simulink library "Animation_Lib"  (R2022b)
settings: Solver=ode45  StartTime=0.0  StopTime=10.0  RelTol=1e-3  EnableMultiTasking=on
undefined symbols (not defined in the file or in its folder): DCT_Param
libraries: vrlib x5, simulink x2, $bdroot x1
Description:
  | Copyright 2014-2022 The MathWorks, Inc.
settings Model: Creator=smiller  LastModifiedBy=smiller
settings SolverCC: AlgebraicLoopSolver=TrustRegion
settings DataIOCC: LimitDataPoints=on  SaveFormat=Array  SignalLoggingSaveFormat=ModelDataLogs  ReturnWorkspaceOutputs=off
settings OptimizationCC: ExpressionDepthLimit=2147483647  LifeSpan=inf
settings DebuggingCC: UnderspecifiedInitializationDetection=Classic  MergeDetectMultiDrivingBlocksExec=none  SolverPrmCheckMsg=warning  FcnCallInpInsideContextMsg=warning  UnconnectedInputMsg=warning  UnconnectedOutputMsg=warning  UnconnectedLineMsg=warning  AllowSymbolicDim=off  StateNameClashWarn=warning  PregeneratedLibrarySubsystemCodeDiagnostic=none  SFUnexpectedBacktrackingDiag=warning  SFNoUnconditionalDefaultTransitionDiag=warning  SFExecutionAtInitializationDiag=none  SFMachineParentedDataDiag=warning  ArithmeticOperatorsInVariantConditions=warning
settings HardwareCC: ProdBitPerPointer=32  ProdBitPerSizeT=32  ProdBitPerPtrDiffT=32  ProdLargestAtomicFloat=None  ProdIntDivRoundTo=Undefined  ProdEndianess=Unspecified  ProdWordSize=32  ProdHWDeviceType=32-bit Generic
settings ModelReferenceCC: EnableRefExpFcnMdlSchedulingChecks=on  PropagateSignalLabelsOutOfModel=off
settings SFSimCC: SimUseLocalCustomCode=off  CustomCodeUndefinedFunction=UseInterfaceOnly
settings RTWCC: RTWUseLocalCustomCode=off  DLArmComputeVersion=19.05
settings CodeAppCC: StateflowObjectComments=on
settings GRTTargetCC: TargetLangStandard=C89/C90 (ANSI)  CombineOutputUpdateFcns=off  GRTInterface=on
settings ConfigComp: CovMetricSettings=dw  CovSaveCumulativeToWorkspaceVar=on  CovSaveSingleToWorkspaceVar=on  CovExternalEMLEnable=off  CovSFcnEnable=off

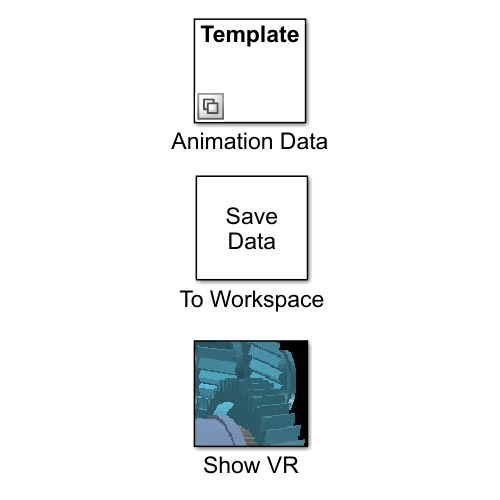
[thumbnail: Simulink's stored preview of the top-level diagram]
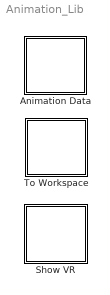
== system Animation_Lib ==
  Animation Data : Subsystem  BlockChoice=Show VR
      settings: TemplateBlock=self  MemberBlocks=Show VR,To Workspace
  Show VR : Subsystem
      mask Display: image(imread('DCT_Animation_Show_VR_IMAGE.jpg'));
  To Workspace : Subsystem
      mask Display: disp('Save\nData');

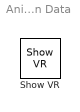
== system Animation_Lib/Animation Data ==
  Show VR : $bdroot/Show VR  SystemSampleTime=-1  VariantActivationTime=update diagram  Latency=0  AutoFrameSizeCalculation=off

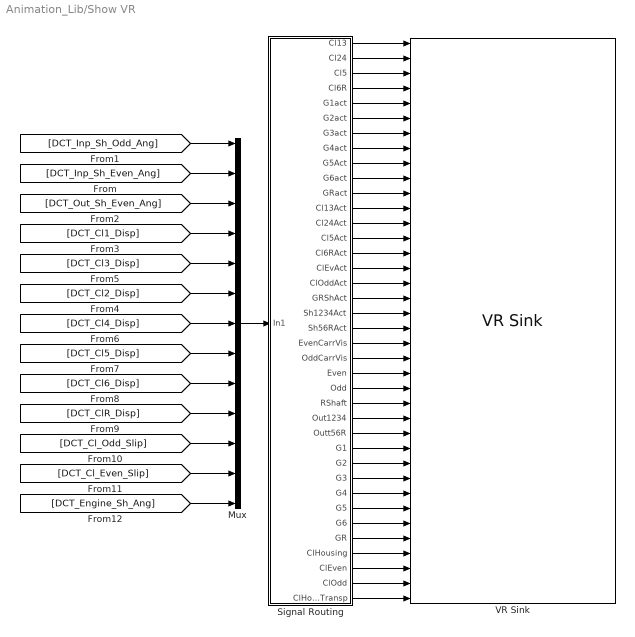
== system Animation_Lib/Show VR ==
  Mux : Mux  Inputs=13
  Signal Routing : Subsystem
  VR Sink : vrlib/VR Sink  InstantiateOnLoad=on  SampleTime=0.1  ViewEnable=on  RemoteChange=off  RemoteView=off  FieldsWritten=DCT.Selector_13_Control.1.1.1.double#DCT.Selector_24_Control.1.1.1.double#DCT.Selector_5_Control.1.1.1.double#DCT.Selector_6R_Control.1.1.1.double#DCT.Gear_1_Active.1.1.1.logical#DCT.Gear_2_Active.1.1.1.logical#DCT.Gear_3_Active.1.1.1.logical#DCT.Gear_4_Active.1.1.1.logical#DCT.Gear_5_Active.1.1.1.logical#DCT.Gear_6_Active.1.1.1.logical#DCT.Gear_R_Active.1.1.1.logical#DCT.Selector_13_Active.1.1.1.logical#DCT.Selector_24_Active.1.1.1.logical#DCT.Selector_5_Active.1.1.1.logical#DCT.Selector_6R_Active.1.1.1.logical#DCT.Clutch_Even_Active.1.1.1.logical#DCT.Clutch_Odd_Active.1.1.1.logical#DCT.Reverse_Shaft_Active.1.1.1.logical#DCT.Shaft_1234_Active.1.1.1.logical#DCT.Shaft_56R_Active.1.1.1.logical#DCT.Clutch_Even_CarrierVis.1.1.1.logical#DCT.Clutch_Odd_CarrierVis.1.1.1.logical#DCT.Input_Shaft_Even_Rot.4.1.1.double#DCT.Input_Shaft_Odd_Rot.4.1.1.double#DCT.Reverse_Shaft_Rot.4.1.1.double#DCT.Output_Shaft_1234_Rot.4.1.1.double#DCT.Output_Shaft_56R_Rot.4.1.1.double#DCT.Gear_1_Rot.4.1.1.double#DCT.Gear_2_Rot.4.1.1.double#DCT.Gear_3_Rot.4.1.1.double#DCT.Gear_4_Rot.4.1.1.double#DCT.Gear_5_Rot.4.1.1.double#DCT.Gear_6_Rot.4.1.1.double#DCT.Gear_R_Rot.4.1.1.double#DCT.Clutch_Driving_Rot.4.1.1.double#DCT.Clutch_Even_Rot.4.1.1.double#DCT.Clutch_Odd_Rot.4.1.1.double#DCT.Clutch_Transparency.1.1.1.double  WorldFileName=DCT_Gearbox_Animation.wrl  WorldDescription=Dual Clutch Transmission  AutoView=off  VideoDimensions=[]  AllowVariableSize=off
  wires:
  [DCT_Inp_Sh_Even_Ang] -> Mux/2
  [DCT_Inp_Sh_Odd_Ang] -> Mux/1
  [DCT_Out_Sh_Even_Ang] -> Mux/3
  [DCT_Cl1_Disp] -> Mux/4
  [DCT_Cl3_Disp] -> Mux/5
  [DCT_Cl2_Disp] -> Mux/6
  [DCT_Cl4_Disp] -> Mux/7
  [DCT_Cl5_Disp] -> Mux/8
  [DCT_Cl6_Disp] -> Mux/9
  [DCT_ClR_Disp] -> Mux/10
  [DCT_Cl_Odd_Slip] -> Mux/11
  [DCT_Cl_Even_Slip] -> Mux/12
  Signal Routing/22(OddCarrVis) -> VR Sink/22
  Signal Routing/21(EvenCarrVis) -> VR Sink/21
  Signal Routing/24(Odd) -> VR Sink/24
  Signal Routing/1(Cl13) -> VR Sink/1
  Signal Routing/26(Out1234) -> VR Sink/26
  Signal Routing/27(Outt56R) -> VR Sink/27
  Signal Routing/28(G1) -> VR Sink/28
  Signal Routing/29(G2) -> VR Sink/29
  Signal Routing/30(G3) -> VR Sink/30
  Signal Routing/31(G4) -> VR Sink/31
  Signal Routing/2(Cl24) -> VR Sink/2
  Signal Routing/5(G1act) -> VR Sink/5
  Signal Routing/7(G3act) -> VR Sink/7
  Signal Routing/6(G2act) -> VR Sink/6
  Signal Routing/8(G4act) -> VR Sink/8
  Signal Routing/3(Cl5) -> VR Sink/3
  Signal Routing/10(G6act) -> VR Sink/10
  Signal Routing/11(GRact) -> VR Sink/11
  Signal Routing/4(Cl6R) -> VR Sink/4
  Signal Routing/32(G5) -> VR Sink/32
  Signal Routing/12(Cl13Act) -> VR Sink/12
  Signal Routing/13(Cl24Act) -> VR Sink/13
  Signal Routing/9(G5Act) -> VR Sink/9
  Signal Routing/14(Cl5Act) -> VR Sink/14
  Signal Routing/15(Cl6RAct) -> VR Sink/15
  Signal Routing/18(GRShAct) -> VR Sink/18
  Signal Routing/16(ClEvAct) -> VR Sink/16
  Signal Routing/17(ClOddAct) -> VR Sink/17
  Signal Routing/19(Sh1234Act) -> VR Sink/19
  Signal Routing/20(Sh56RAct) -> VR Sink/20
  Signal Routing/25(RShaft) -> VR Sink/25
  Signal Routing/23(Even) -> VR Sink/23
  Signal Routing/33(G6) -> VR Sink/33
  Signal Routing/34(GR) -> VR Sink/34
  Signal Routing/35(ClHousing) -> VR Sink/35
  Signal Routing/36(ClEven) -> VR Sink/36
  Mux/1 -> Signal Routing/1(In1)
  [DCT_Engine_Sh_Ang] -> Mux/13
  Signal Routing/37(ClOdd) -> VR Sink/37
  Signal Routing/38(ClHousTransp) -> VR Sink/38

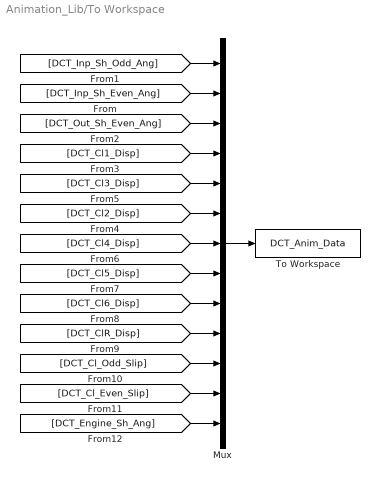
== system Animation_Lib/To Workspace ==
  Mux : Mux  Inputs=13
  To Workspace : ToWorkspace  VariableName=DCT_Anim_Data  SaveFormat=Structure With Time  SampleTime=-1
  wires:
  [DCT_Cl_Even_Slip] -> Mux/12
  [DCT_Cl_Odd_Slip] -> Mux/11
  [DCT_ClR_Disp] -> Mux/10
  [DCT_Cl6_Disp] -> Mux/9
  [DCT_Cl5_Disp] -> Mux/8
  [DCT_Cl4_Disp] -> Mux/7
  [DCT_Cl2_Disp] -> Mux/6
  [DCT_Cl3_Disp] -> Mux/5
  [DCT_Cl1_Disp] -> Mux/4
  [DCT_Out_Sh_Even_Ang] -> Mux/3
  [DCT_Inp_Sh_Odd_Ang] -> Mux/1
  [DCT_Inp_Sh_Even_Ang] -> Mux/2
  Mux/1 -> To Workspace/1
  [DCT_Engine_Sh_Ang] -> Mux/13

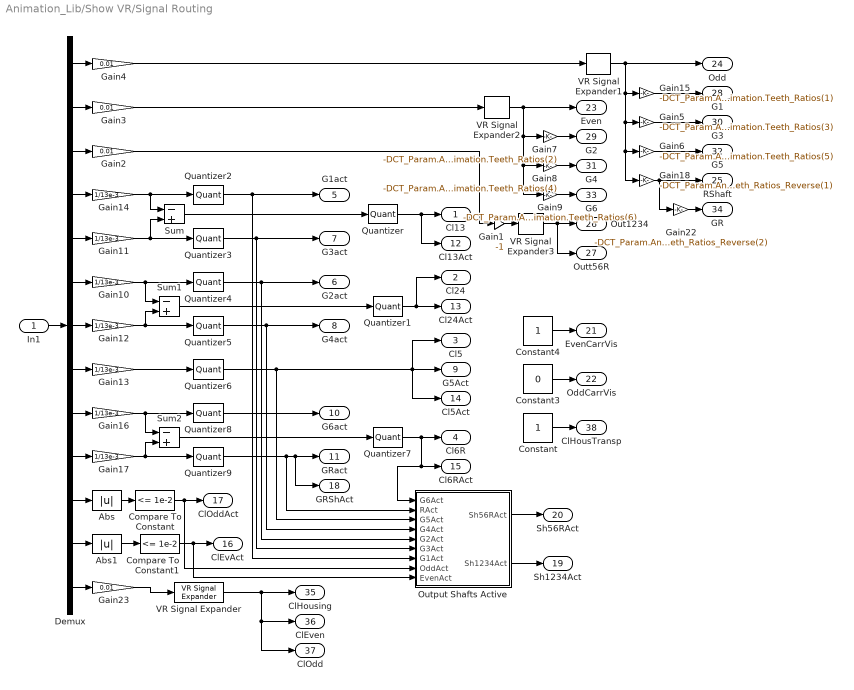
== system Animation_Lib/Show VR/Signal Routing ==
  In1 : Inport
  Abs : Abs  SaturateOnIntegerOverflow=off
  Abs1 : Abs  SaturateOnIntegerOverflow=off
  Compare To Constant : simulink/Logic and Bit Operations/Compare To Constant  relop=<=  const=1e-2  OutDataTypeStr=uint8
  Compare To Constant1 : simulink/Logic and Bit Operations/Compare To Constant  relop=<=  const=1e-2  OutDataTypeStr=uint8
  Constant : Constant
  Constant3 : Constant  Value=0
  Constant4 : Constant
  Demux : Demux  Outputs=13
  Gain1 : Gain  Gain=-1
  Gain{10..14,16..17} (7 alike) : Gain  Gain=1/13e-3
  Gain15 : Gain  Gain=-DCT_Param.Animation.Teeth_Ratios(1)
  Gain18 : Gain  Gain=-DCT_Param.Animation.Teeth_Ratios_Reverse(1)
  Gain{2..4,23} (4 alike) : Gain  Gain=0.01
  Gain22 : Gain  Gain=-DCT_Param.Animation.Teeth_Ratios_Reverse(2)
  Gain5 : Gain  Gain=-DCT_Param.Animation.Teeth_Ratios(3)
  Gain6 : Gain  Gain=-DCT_Param.Animation.Teeth_Ratios(5)
  Gain7 : Gain  Gain=-DCT_Param.Animation.Teeth_Ratios(2)
  Gain8 : Gain  Gain=-DCT_Param.Animation.Teeth_Ratios(4)
  Gain9 : Gain  Gain=-DCT_Param.Animation.Teeth_Ratios(6)
  Output Shafts Active : Subsystem
  Quantizer{,1..9} (10 alike) : Quantizer  QuantizationInterval=0.1
  Sum : Sum  Inputs=-+
  Sum1 : Sum  Inputs=-+
  Sum2 : Sum  Inputs=-+
  VR Signal Expander{,1..3} (4 alike) : vrlib/VR Signal Expander  outwidth=4  outidx=[4]
  Cl13 : Outport  VectorParamsAs1DForOutWhenUnconnected=off
  Cl24 : Outport  Port=2  VectorParamsAs1DForOutWhenUnconnected=off
  Cl5 : Outport  Port=3  VectorParamsAs1DForOutWhenUnconnected=off
  Cl6R : Outport  Port=4  VectorParamsAs1DForOutWhenUnconnected=off
  G1act : Outport  Port=5  VectorParamsAs1DForOutWhenUnconnected=off
  G2act : Outport  Port=6  VectorParamsAs1DForOutWhenUnconnected=off
  G3act : Outport  Port=7  VectorParamsAs1DForOutWhenUnconnected=off
  G4act : Outport  Port=8  VectorParamsAs1DForOutWhenUnconnected=off
  G5Act : Outport  Port=9  VectorParamsAs1DForOutWhenUnconnected=off
  G6act : Outport  Port=10  VectorParamsAs1DForOutWhenUnconnected=off
  GRact : Outport  Port=11  VectorParamsAs1DForOutWhenUnconnected=off
  Cl13Act : Outport  Port=12  VectorParamsAs1DForOutWhenUnconnected=off
  Cl24Act : Outport  Port=13  VectorParamsAs1DForOutWhenUnconnected=off
  Cl5Act : Outport  Port=14  VectorParamsAs1DForOutWhenUnconnected=off
  Cl6RAct : Outport  Port=15  VectorParamsAs1DForOutWhenUnconnected=off
  ClEvAct : Outport  Port=16  VectorParamsAs1DForOutWhenUnconnected=off
  ClOddAct : Outport  Port=17  VectorParamsAs1DForOutWhenUnconnected=off
  GRShAct : Outport  Port=18  VectorParamsAs1DForOutWhenUnconnected=off
  Sh1234Act : Outport  Port=19  VectorParamsAs1DForOutWhenUnconnected=off
  Sh56RAct : Outport  Port=20  VectorParamsAs1DForOutWhenUnconnected=off
  EvenCarrVis : Outport  Port=21  VectorParamsAs1DForOutWhenUnconnected=off
  OddCarrVis : Outport  Port=22  VectorParamsAs1DForOutWhenUnconnected=off
  Even : Outport  Port=23  VectorParamsAs1DForOutWhenUnconnected=off
  Odd : Outport  Port=24  VectorParamsAs1DForOutWhenUnconnected=off
  RShaft : Outport  Port=25  VectorParamsAs1DForOutWhenUnconnected=off
  Out1234 : Outport  Port=26  VectorParamsAs1DForOutWhenUnconnected=off
  Outt56R : Outport  Port=27  VectorParamsAs1DForOutWhenUnconnected=off
  G1 : Outport  Port=28  VectorParamsAs1DForOutWhenUnconnected=off
  G2 : Outport  Port=29  VectorParamsAs1DForOutWhenUnconnected=off
  G3 : Outport  Port=30  VectorParamsAs1DForOutWhenUnconnected=off
  G4 : Outport  Port=31  VectorParamsAs1DForOutWhenUnconnected=off
  G5 : Outport  Port=32  VectorParamsAs1DForOutWhenUnconnected=off
  G6 : Outport  Port=33  VectorParamsAs1DForOutWhenUnconnected=off
  GR : Outport  Port=34  VectorParamsAs1DForOutWhenUnconnected=off
  ClHousing : Outport  Port=35  VectorParamsAs1DForOutWhenUnconnected=off
  ClEven : Outport  Port=36  VectorParamsAs1DForOutWhenUnconnected=off
  ClOdd : Outport  Port=37  VectorParamsAs1DForOutWhenUnconnected=off
  ClHousTransp : Outport  Port=38  VectorParamsAs1DForOutWhenUnconnected=off
  wires:
  Demux/1 -> Gain4/1
  Demux/2 -> Gain3/1
  In1/1 -> Demux/1
  Demux/3 -> Gain2/1
  Quantizer/1 -> Cl13/1, Cl13Act/1
  Gain2/1 -> Gain1/1
  Gain3/1 -> VR Signal Expander2/1
  Gain4/1 -> VR Signal Expander1/1
  Demux/5 -> Gain11/1
  Sum/1 -> Quantizer/1
  Sum1/1 -> Quantizer1/1
  Quantizer1/1 -> Cl24/1, Cl24Act/1
  Demux/7 -> Gain12/1
  Demux/6 -> Gain10/1
  Demux/4 -> Gain14/1
  Gain14/1 -> Sum/1, Quantizer2/1
  Gain11/1 -> Sum/2, Quantizer3/1
  Quantizer2/1 -> G1act/1, Output Shafts Active/7(G1Act)
  Quantizer3/1 -> G3act/1, Output Shafts Active/6(G3Act)
  Gain10/1 -> Sum1/1, Quantizer4/1
  Gain12/1 -> Sum1/2, Quantizer5/1
  Quantizer4/1 -> G2act/1, Output Shafts Active/5(G2Act)
  Quantizer5/1 -> G4act/1, Output Shafts Active/4(G4Act)
  Demux/8 -> Gain13/1
  Quantizer6/1 -> Cl5/1, G5Act/1, Cl5Act/1, Output Shafts Active/3(G5Act)
  Gain13/1 -> Quantizer6/1
  Sum2/1 -> Quantizer7/1
  Quantizer7/1 -> Cl6R/1, Cl6RAct/1, Output Shafts Active/1(G6Act)
  Gain16/1 -> Quantizer8/1, Sum2/1
  Gain17/1 -> Quantizer9/1, Sum2/2
  Quantizer8/1 -> G6act/1
  Quantizer9/1 -> GRact/1, GRShAct/1, Output Shafts Active/2(RAct)
  Demux/9 -> Gain16/1
  Demux/10 -> Gain17/1
  VR Signal Expander/1 -> ClHousing/1, ClEven/1, ClOdd/1
  Constant/1 -> ClHousTransp/1
  Demux/11 -> Abs/1
  Abs/1 -> Compare To Constant/1
  Abs1/1 -> Compare To Constant1/1
  Demux/12 -> Abs1/1
  Compare To Constant1/1 -> ClEvAct/1, Output Shafts Active/9(EvenAct)
  Compare To Constant/1 -> ClOddAct/1, Output Shafts Active/8(OddAct)
  Output Shafts Active/1(Sh56RAct) -> Sh56RAct/1
  Output Shafts Active/2(Sh1234Act) -> Sh1234Act/1
  Constant3/1 -> OddCarrVis/1
  Constant4/1 -> EvenCarrVis/1
  Demux/13 -> Gain23/1
  Gain23/1 -> VR Signal Expander/1
  Gain22/1 -> GR/1
  Gain18/1 -> RShaft/1, Gain22/1
  Gain9/1 -> G6/1
  Gain8/1 -> G4/1
  Gain7/1 -> G2/1
  Gain6/1 -> G5/1
  Gain5/1 -> G3/1
  Gain15/1 -> G1/1
  VR Signal Expander3/1 -> Out1234/1, Outt56R/1
  Gain1/1 -> VR Signal Expander3/1
  VR Signal Expander2/1 -> Even/1, Gain7/1, Gain8/1, Gain9/1
  VR Signal Expander1/1 -> Odd/1, Gain15/1, Gain5/1, Gain6/1, Gain18/1

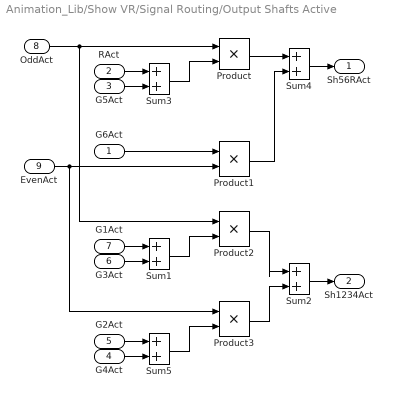
== system Animation_Lib/Show VR/Signal Routing/Output Shafts Active ==
  G6Act : Inport
  RAct : Inport  Port=2
  G5Act : Inport  Port=3
  G4Act : Inport  Port=4
  G2Act : Inport  Port=5
  G3Act : Inport  Port=6
  G1Act : Inport  Port=7
  OddAct : Inport  Port=8
  EvenAct : Inport  Port=9
  Product{,1..3} (4 alike) : Product  RndMeth=Zero
  Sum{1..5} (5 alike) : Sum
  Sh56RAct : Outport  VectorParamsAs1DForOutWhenUnconnected=off
  Sh1234Act : Outport  Port=2  VectorParamsAs1DForOutWhenUnconnected=off
  wires:
  Product/1 -> Sum4/1
  Product1/1 -> Sum4/2
  Sum4/1 -> Sh56RAct/1
  RAct/1 -> Sum3/1
  G5Act/1 -> Sum3/2
  OddAct/1 -> Product2/1, Product/1
  G6Act/1 -> Product1/1
  EvenAct/1 -> Product1/2, Product3/1
  G1Act/1 -> Sum1/1
  G3Act/1 -> Sum1/2
  G2Act/1 -> Sum5/1
  G4Act/1 -> Sum5/2
  Sum1/1 -> Product2/2
  Product2/1 -> Sum2/1
  Sum2/1 -> Sh1234Act/1
  Sum5/1 -> Product3/2
  Product3/1 -> Sum2/2
  Sum3/1 -> Product/2
